simulink model "Pacemaker_Assignment2_group33_Final"  (R2020a)
settings: Solver=FixedStepAuto  StartTime=0.0  StopTime=10.0  FixedStep=1e-3  RelTol=1e-3  EnableMultiTasking=on
undefined symbols (not defined in the file): A0, A1, D0, D1, D10, D11, D12, D13, D2, D3, D4, D5, D6, D7, D8, D9, magnitude, PTA0, PTA1, PTA2, PTB2, PTB23, PTB3, PTB9, PTC16, PTC17, PTC2, PTC3, PTC4, PTD0, PTD1, PTD2, PTD3
libraries: frdmk64flib x22, etargetslib x16, dspstat3 x1
settings Model: ExtModeTrigDuration=5  Creator=sxj  LastModifiedBy=sxj
settings OptimizationCC: EnhancedBackFolding=on  PassReuseOutputArgsAs=Individual arguments  ZeroExternalMemoryAtStartup=off  ZeroInternalMemoryAtStartup=off  MaxStackSize=64  OptimizeBlockOrder=speed  DifferentSizesBufferReuse=on  OptimizationCustomize=off  EfficientTunableParamExpr=on
settings DebuggingCC: ParameterTunabilityLossMsg=error
settings HardwareCC: ProdBitPerPointer=32  ProdBitPerSizeT=32  ProdBitPerPtrDiffT=32  ProdLargestAtomicInteger=Long  ProdLargestAtomicFloat=Double  ProdWordSize=32  ProdHWDeviceType=ARM Compatible->ARM Cortex
settings SFSimCC: MATLABDynamicMemAlloc=off
settings RTWCC: SystemTargetFile=ert.tlc  HardwareBoard=NXP FRDM-K64F  TemplateMakefile=ert_default_tmf  Toolchain=GNU Tools for ARM Embedded Processors
settings CodeAppCC: ForceParamTrailComments=on  IgnoreCustomStorageClasses=off  OperatorAnnotations=on  SimulinkDataObjDesc=on  SFDataObjDesc=on  InsertBlockDesc=on

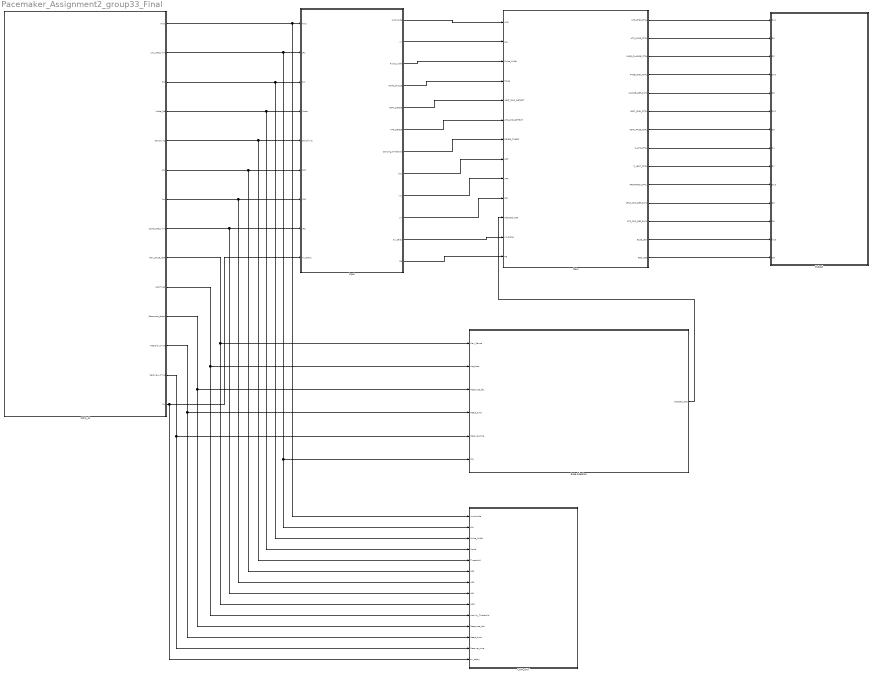
== system Pacemaker_Assignment2_group33_Final ==
  COM_IN : Subsystem
  COM_OUT : Subsystem
  Input : Subsystem
  Main : Stateflow chart  TreatAsAtomicUnit=on
  Output : Subsystem
  Rate Adaption : Subsystem
  wires:
  Input/1(Amplitude) -> Main/1(AMP)
  Input/2(lrl) -> Main/2(LRL)
  Input/3(Pulse_width) -> Main/3(Pulse_Width)
  Input/4(Mode_choose) -> Main/4(Mode)
  Input/5(VENT_SENSE) -> Main/5(VENT_CMP_DETECT)
  Input/6(ATR_SENSE) -> Main/6(ATR_CMP_DETECT)
  Input/7(Sensing_Threshold) -> Main/7(SENSE_THRES)
  Main/1(ATR_GND_CTRL) -> Output/1(D11)
  Main/2(ATR_PACE_CTRL) -> Output/2(D8)
  Main/3(PACE_CHARGE_CTRL) -> Output/3(D2)
  Main/4(PACE_GND_CTRL) -> Output/4(D10)
  Main/5(PACING_REF_PWM) -> Output/5(D5)
  Main/6(VENT_GND_CTRL) -> Output/6(D12)
  Main/7(VENT_PACE_CTRL) -> Output/7(D9)
  Main/8(Z_ATR_CTRL) -> Output/8(D4)
  Main/9(Z_VENT_CTRL) -> Output/9(D7)
  Main/10(FRONTEND_CTRL) -> Output/10(D13)
  Main/11(VENT_CMP_REF_PWM) -> Output/11(D3)
  Main/12(ATR_CMP_REF_PWM) -> Output/12(D6)
  Main/13(BLUE_LED) -> Output/13(blue)
  Main/14(RED_LED) -> Output/14(red)
  Input/8(arp) -> Main/8(ARP)
  Input/9(vrp) -> Main/9(VRP)
  Input/10(url) -> Main/10(URL)
  Rate Adaption/1(Adapted_rate) -> Main/11(Adapted_rate)
  COM_IN/1(Amp) -> COM_OUT/1(Amplitude), Input/1(Amp)
  COM_IN/2(Low_rate_limit) -> COM_OUT/2(LRL), Rate Adaption/6(LRL), Input/2(LRL)
  COM_IN/3(PW) -> COM_OUT/3(Pulse_Width), Input/3(PW)
  COM_IN/4(Mode_Sel) -> COM_OUT/4(Mode), Input/4(Mode)
  COM_IN/5(Sensitivity) -> COM_OUT/5(Threshold), Input/5(Sensitivity)
  COM_IN/6(Arp) -> COM_OUT/6(ARP), Input/6(ARP)
  COM_IN/7(Vrp) -> COM_OUT/7(VRP), Input/7(VRP)
  COM_IN/8(Upper_rate_limit) -> COM_OUT/8(URL), Input/8(URL)
  COM_IN/9(Max_sense_rate) -> COM_OUT/9(MSR), Rate Adaption/1(Max_Sense)
  COM_IN/10(Act_Thres) -> COM_OUT/10(Activity_Threshold), Rate Adaption/2(Act_thres)
  COM_IN/11(Response_factor) -> COM_OUT/11(Response_Fac), Rate Adaption/3(Response_fac)
  COM_IN/12(Reaction_Time) -> COM_OUT/12(React_time), Rate Adaption/4(React_time)
  COM_IN/13(Recovery_Time) -> COM_OUT/13(Recover_time), Rate Adaption/5(Recover_time)
  COM_IN/14(AV) -> COM_OUT/14(av_delay), Input/9(AV_Delay)
  Input/11(av_delay) -> Main/12(AV_Delay)
  Input/12(PB) -> Main/13(PB)

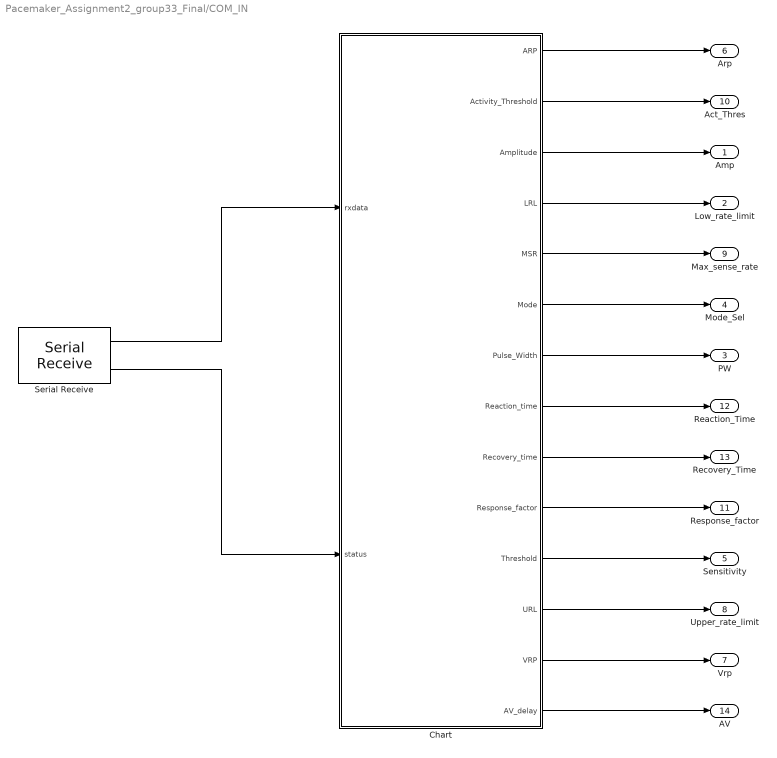
== system Pacemaker_Assignment2_group33_Final/COM_IN ==
  Chart : Stateflow chart  TreatAsAtomicUnit=on
  Serial Receive : frdmk64flib/Serial Receive  SCIModule=0  Baudrate=uint32(9600)  Parity=None  StopBits=1  HardwareFlowControl=None  ByteOrder=LittleEndian  DataType=uint8  DataLength=36  BlockingMode=off  OutputStatus=on  SampleTime=-1
  Amp : Outport
  Low_rate_limit : Outport  Port=2  OutDataTypeStr=uint16
  PW : Outport  Port=3
  Mode_Sel : Outport  Port=4
  Sensitivity : Outport  Port=5
  Arp : Outport  Port=6
  Vrp : Outport  Port=7
  Upper_rate_limit : Outport  Port=8
  Max_sense_rate : Outport  Port=9
  Act_Thres : Outport  Port=10
  Response_factor : Outport  Port=11
  Reaction_Time : Outport  Port=12
  Recovery_Time : Outport  Port=13
  AV : Outport  Port=14
  wires:
  Serial Receive/1 -> Chart/1(rxdata)
  Chart/1(ARP) -> Arp/1
  Chart/2(Activity_Threshold) -> Act_Thres/1
  Chart/3(Amplitude) -> Amp/1
  Chart/4(LRL) -> Low_rate_limit/1
  Chart/5(MSR) -> Max_sense_rate/1
  Chart/6(Mode) -> Mode_Sel/1
  Chart/7(Pulse_Width) -> PW/1
  Chart/8(Reaction_time) -> Reaction_Time/1
  Chart/9(Recovery_time) -> Recovery_Time/1
  Chart/10(Response_factor) -> Response_factor/1
  Chart/11(Threshold) -> Sensitivity/1
  Chart/12(URL) -> Upper_rate_limit/1
  Chart/13(VRP) -> Vrp/1
  Serial Receive/2 -> Chart/2(status)
  Chart/14(AV_delay) -> AV/1

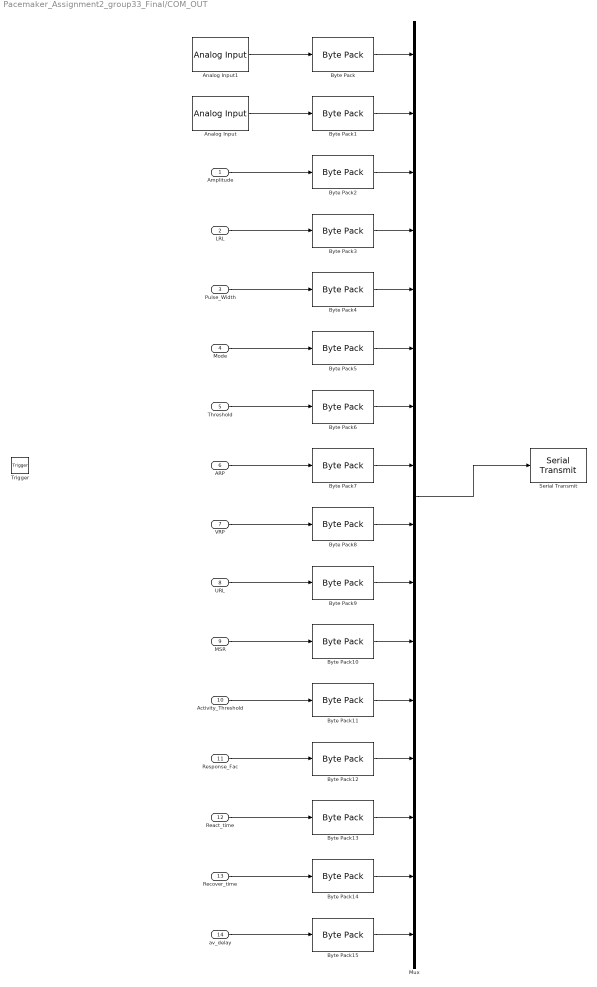
== system Pacemaker_Assignment2_group33_Final/COM_OUT ==
  Amplitude : Inport
  LRL : Inport  Port=2
  Pulse_Width : Inport  Port=3
  Mode : Inport  Port=4
  Threshold : Inport  Port=5
  ARP : Inport  Port=6
  VRP : Inport  Port=7
  URL : Inport  Port=8
  MSR : Inport  Port=9
  Activity_Threshold : Inport  Port=10
  Response_Fac : Inport  Port=11
  React_time : Inport  Port=12
  Recover_time : Inport  Port=13
  av_delay : Inport  Port=14
  Trigger : TriggerPort  TriggerType=function-call  IsSimulinkFunction=on  FunctionName=send_params  VariantControl=Variant  PortDimensions=1
  Analog Input : frdmk64flib/Analog Input  Whichpin=PTB3 (A1)  SampleTime=-1
  Analog Input1 : frdmk64flib/Analog Input  Whichpin=PTB2 (A0)  SampleTime=-1
  Byte Pack : etargetslib/Byte Pack  datatypes={'double'}  byteAlign=1
  Byte Pack1 : etargetslib/Byte Pack  datatypes={'double'}  byteAlign=1
  Byte Pack{2..3,5..6,9..10,12..14} (9 alike) : etargetslib/Byte Pack  datatypes={'uint16'}  byteAlign=1
  Byte Pack{4,7..8,11,15} (5 alike) : etargetslib/Byte Pack  datatypes={'single'}  byteAlign=1
  Mux : Mux  Inputs=16
  Serial Transmit : frdmk64flib/Serial Transmit  SCIModule=0  Baudrate=uint32(9600)  Parity=None  StopBits=1  HardwareFlowControl=None  ByteOrder=LittleEndian  BlockingMode=on  OutputStatus=off
  wires:
  Analog Input/1 -> Byte Pack1/1
  Byte Pack/1 -> Mux/1
  Mux/1 -> Serial Transmit/1
  Analog Input1/1 -> Byte Pack/1
  Byte Pack1/1 -> Mux/2
  LRL/1 -> Byte Pack3/1
  Amplitude/1 -> Byte Pack2/1
  Pulse_Width/1 -> Byte Pack4/1
  Mode/1 -> Byte Pack5/1
  Threshold/1 -> Byte Pack6/1
  ARP/1 -> Byte Pack7/1
  VRP/1 -> Byte Pack8/1
  URL/1 -> Byte Pack9/1
  MSR/1 -> Byte Pack10/1
  Activity_Threshold/1 -> Byte Pack11/1
  Response_Fac/1 -> Byte Pack12/1
  React_time/1 -> Byte Pack13/1
  Recover_time/1 -> Byte Pack14/1
  Byte Pack2/1 -> Mux/3
  Byte Pack3/1 -> Mux/4
  Byte Pack4/1 -> Mux/5
  Byte Pack5/1 -> Mux/6
  Byte Pack6/1 -> Mux/7
  Byte Pack7/1 -> Mux/8
  Byte Pack8/1 -> Mux/9
  Byte Pack9/1 -> Mux/10
  Byte Pack10/1 -> Mux/11
  Byte Pack11/1 -> Mux/12
  Byte Pack12/1 -> Mux/13
  Byte Pack13/1 -> Mux/14
  Byte Pack14/1 -> Mux/15
  av_delay/1 -> Byte Pack15/1
  Byte Pack15/1 -> Mux/16

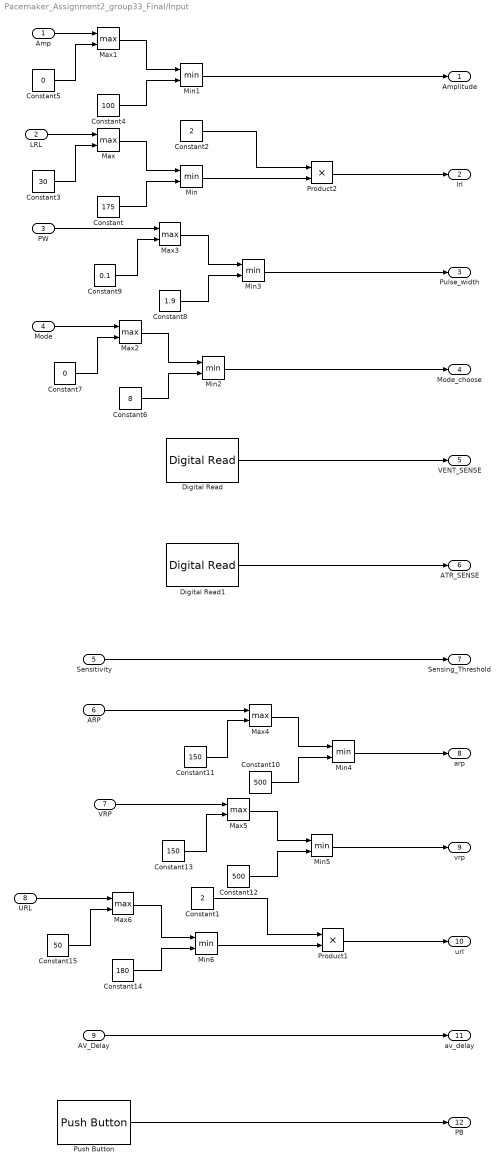
== system Pacemaker_Assignment2_group33_Final/Input ==
  Amp : Inport
  LRL : Inport  Port=2
  PW : Inport  Port=3
  Mode : Inport  Port=4
  Sensitivity : Inport  Port=5
  ARP : Inport  Port=6
  VRP : Inport  Port=7
  URL : Inport  Port=8
  AV_Delay : Inport  Port=9
  Constant : Constant  Value=175
  Constant1 : Constant  Value=2
  Constant10 : Constant  Value=500
  Constant11 : Constant  Value=150
  Constant12 : Constant  Value=500
  Constant13 : Constant  Value=150
  Constant14 : Constant  Value=180
  Constant15 : Constant  Value=50
  Constant2 : Constant  Value=2
  Constant3 : Constant  Value=30
  Constant4 : Constant  Value=100
  Constant5 : Constant  Value=0
  Constant6 : Constant  Value=8
  Constant7 : Constant  Value=0
  Constant8 : Constant  Value=1.9
  Constant9 : Constant  Value=0.1
  Digital Read : frdmk64flib/Digital Read  Whichpin=PTC17 (D1)  SampleTime=-1
  Digital Read1 : frdmk64flib/Digital Read  Whichpin=PTC16 (D0)  SampleTime=-1
  Max{,3..5} (4 alike) : MinMax  Function=max  Inputs=2  OutDataTypeStr=single
  Max1 : MinMax  Function=max  Inputs=2  OutDataTypeStr=uint16
  Max2 : MinMax  Function=max  Inputs=2  OutDataTypeStr=uint16
  Max6 : MinMax  Function=max  Inputs=2
  Min{,3..5} (4 alike) : MinMax  Inputs=2  OutDataTypeStr=single
  Min1 : MinMax  Inputs=2  OutDataTypeStr=uint16
  Min2 : MinMax  Inputs=2  OutDataTypeStr=uint16
  Min6 : MinMax  Inputs=2
  Product1 : Product  OutDataTypeStr=uint16
  Product2 : Product  OutDataTypeStr=single
  Push Button : frdmk64flib/Push Button  Whichswitch=SW2  SampleTime1=-1
  Amplitude : Outport
  lrl : Outport  Port=2
  Pulse_width : Outport  Port=3
  Mode_choose : Outport  Port=4
  VENT_SENSE : Outport  Port=5
  ATR_SENSE : Outport  Port=6
  Sensing_Threshold : Outport  Port=7
  arp : Outport  Port=8
  vrp : Outport  Port=9
  url : Outport  Port=10
  av_delay : Outport  Port=11
  PB : Outport  Port=12
  wires:
  Digital Read/1 -> VENT_SENSE/1
  Digital Read1/1 -> ATR_SENSE/1
  Sensitivity/1 -> Sensing_Threshold/1
  Product1/1 -> url/1
  Constant1/1 -> Product1/1
  Constant2/1 -> Product2/1
  Product2/1 -> lrl/1
  AV_Delay/1 -> av_delay/1
  Push Button/1 -> PB/1
  Constant/1 -> Min/2
  Max/1 -> Min/1
  Constant3/1 -> Max/2
  Min/1 -> Product2/2
  Constant4/1 -> Min1/2
  Constant5/1 -> Max1/2
  Max1/1 -> Min1/1
  Amp/1 -> Max1/1
  LRL/1 -> Max/1
  Min1/1 -> Amplitude/1
  Constant6/1 -> Min2/2
  Constant7/1 -> Max2/2
  Max2/1 -> Min2/1
  Min2/1 -> Mode_choose/1
  Mode/1 -> Max2/1
  Constant8/1 -> Min3/2
  Constant9/1 -> Max3/2
  Max3/1 -> Min3/1
  PW/1 -> Max3/1
  Min3/1 -> Pulse_width/1
  Constant10/1 -> Min4/2
  Constant11/1 -> Max4/2
  Max4/1 -> Min4/1
  Min4/1 -> arp/1
  ARP/1 -> Max4/1
  Constant12/1 -> Min5/2
  Constant13/1 -> Max5/2
  Max5/1 -> Min5/1
  Min5/1 -> vrp/1
  VRP/1 -> Max5/1
  Constant14/1 -> Min6/2
  Constant15/1 -> Max6/2
  Max6/1 -> Min6/1
  Min6/1 -> Product1/2
  URL/1 -> Max6/1

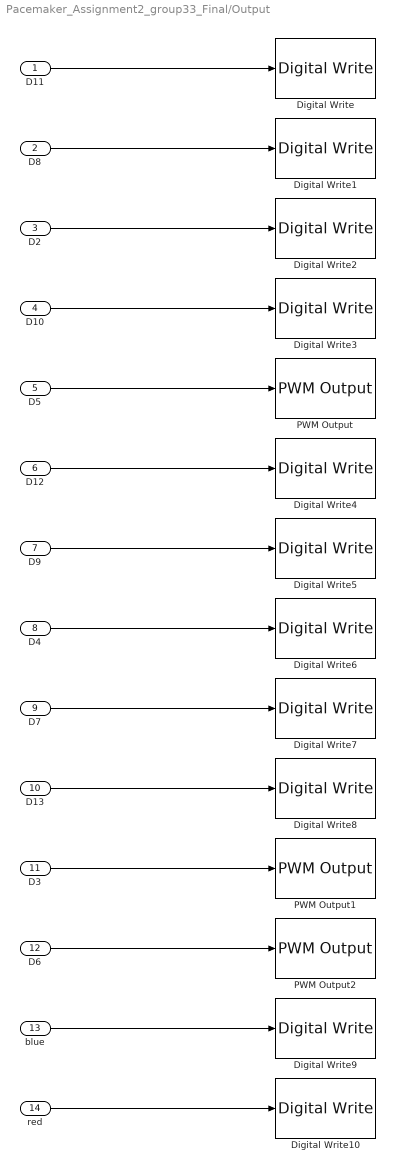
== system Pacemaker_Assignment2_group33_Final/Output ==
  D11 : Inport
  D8 : Inport  Port=2
  D2 : Inport  Port=3
  D10 : Inport  Port=4
  D5 : Inport  Port=5
  D12 : Inport  Port=6
  D9 : Inport  Port=7
  D4 : Inport  Port=8
  D7 : Inport  Port=9
  D13 : Inport  Port=10
  D3 : Inport  Port=11
  D6 : Inport  Port=12
  blue : Inport  Port=13
  red : Inport  Port=14
  Digital Write : frdmk64flib/Digital Write  Whichpin=PTD2 (D11)
  Digital Write1 : frdmk64flib/Digital Write  Whichpin=PTA0 (D8)
  Digital Write10 : frdmk64flib/Digital Write  Whichpin=RED_LED
  Digital Write2 : frdmk64flib/Digital Write  Whichpin=PTB9 (D2)
  Digital Write3 : frdmk64flib/Digital Write  Whichpin=PTD0 (D10)
  Digital Write4 : frdmk64flib/Digital Write  Whichpin=PTD3 (D12)
  Digital Write5 : frdmk64flib/Digital Write  Whichpin=PTC4 (D9)
  Digital Write6 : frdmk64flib/Digital Write  Whichpin=PTB23 (D4)
  Digital Write7 : frdmk64flib/Digital Write  Whichpin=PTC3 (D7)
  Digital Write8 : frdmk64flib/Digital Write  Whichpin=PTD1 (D13)
  Digital Write9 : frdmk64flib/Digital Write  Whichpin=BLUE_LED
  PWM Output : frdmk64flib/PWM Output  Whichpin=PTA2 (D5)  InitialFrequency=2000  InitialDutyCycle=0
  PWM Output1 : frdmk64flib/PWM Output  Whichpin=PTA1 (D3)  InitialFrequency=2000  InitialDutyCycle=0
  PWM Output2 : frdmk64flib/PWM Output  Whichpin=PTC2 (D6)  InitialFrequency=2000  InitialDutyCycle=0
  wires:
  D11/1 -> Digital Write/1
  D8/1 -> Digital Write1/1
  D2/1 -> Digital Write2/1
  D10/1 -> Digital Write3/1
  D5/1 -> PWM Output/1
  D12/1 -> Digital Write4/1
  D9/1 -> Digital Write5/1
  D4/1 -> Digital Write6/1
  D7/1 -> Digital Write7/1
  D13/1 -> Digital Write8/1
  D3/1 -> PWM Output1/1
  D6/1 -> PWM Output2/1
  blue/1 -> Digital Write9/1
  red/1 -> Digital Write10/1

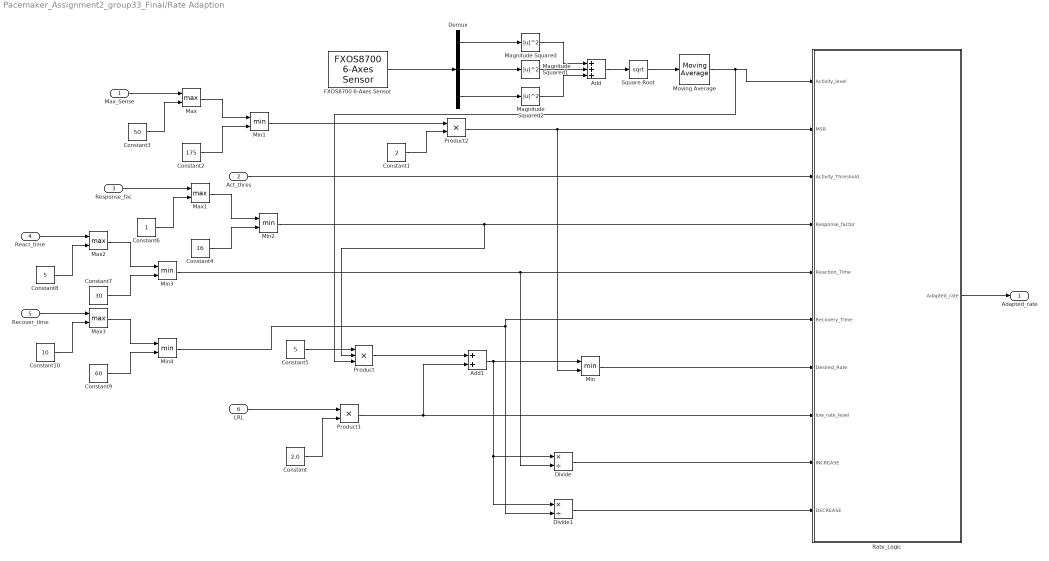
== system Pacemaker_Assignment2_group33_Final/Rate Adaption ==
  Max_Sense : Inport
  Act_thres : Inport  Port=2
  Response_fac : Inport  Port=3
  React_time : Inport  Port=4
  Recover_time : Inport  Port=5
  LRL : Inport  Port=6  OutDataTypeStr=uint16
  Add : Sum  Inputs=+++
  Add1 : Sum
  Constant : Constant  Value=2.0
  Constant1 : Constant  Value=2
  Constant10 : Constant  Value=10
  Constant2 : Constant  Value=175
  Constant3 : Constant  Value=50
  Constant4 : Constant  Value=16
  Constant5 : Constant  Value=5
  Constant6 : Constant
  Constant7 : Constant  Value=30
  Constant8 : Constant  Value=5
  Constant9 : Constant  Value=60
  Demux : Demux  Outputs=3
  Divide : Product  Inputs=*/
  Divide1 : Product  Inputs=*/
  FXOS8700 6-Axes Sensor : frdmk64flib/FXOS8700 6-Axes Sensor  Activesensor=Accelerometer only  ODR=800Hz  HybridODR=400Hz  Accelfullrange=-4g to +4g  SampleTime=-1
  Magnitude Squared : Math  Operator=magnitude^2  SaturateOnIntegerOverflow=on
  Magnitude Squared1 : Math  Operator=magnitude^2  SaturateOnIntegerOverflow=on
  Magnitude Squared2 : Math  Operator=magnitude^2  SaturateOnIntegerOverflow=on
  Max{,1..3} (4 alike) : MinMax  Function=max  Inputs=2  OutDataTypeStr=uint16
  Min : MinMax  Inputs=2
  Min{1..4} (4 alike) : MinMax  Inputs=2  OutDataTypeStr=uint16
  Moving Average : dspstat3/Moving Average  Method=Sliding window  ForgettingFactorPort=off  SpecifyWindowLength=on  WindowLength=100  ForgettingFactor=0.9  SimulateUsing=Code generation
  Product : Product  Inputs=3
  Product1 : Product  OutDataTypeStr=double
  Product2 : Product  OutDataTypeStr=uint8
  Rate_Logic : Stateflow chart  TreatAsAtomicUnit=on
  Square Root : Sqrt  SaturateOnIntegerOverflow=on
  Adapted_rate : Outport
  wires:
  Demux/1 -> Magnitude Squared/1
  Magnitude Squared1/1 -> Add/2
  Add/1 -> Square Root/1
  FXOS8700 6-Axes Sensor/1 -> Demux/1
  Demux/2 -> Magnitude Squared1/1
  Demux/3 -> Magnitude Squared2/1
  Magnitude Squared/1 -> Add/1
  Magnitude Squared2/1 -> Add/3
  Square Root/1 -> Moving Average/1
  Min2/1 -> Product/2, Rate_Logic/4(Response_factor)
  Min3/1 -> Rate_Logic/5(Reaction_Time), Divide/2
  Min4/1 -> Rate_Logic/6(Recovery_Time), Divide1/2
  Moving Average/1 -> Product/3, Rate_Logic/1(Activity_level)
  Product/1 -> Add1/1
  Product1/1 -> Add1/2, Rate_Logic/8(low_rate_level)
  Add1/1 -> Divide1/1, Divide/1, Min/1
  Min/1 -> Rate_Logic/7(Desired_Rate)
  Divide/1 -> Rate_Logic/9(INCREASE)
  Rate_Logic/1(Adapted_rate) -> Adapted_rate/1
  Constant5/1 -> Product/1
  Divide1/1 -> Rate_Logic/10(DECREASE)
  LRL/1 -> Product1/1
  Product2/1 -> Min/2, Rate_Logic/2(MSR)
  Act_thres/1 -> Rate_Logic/3(Activity_Threshold)
  Constant/1 -> Product1/2
  Constant1/1 -> Product2/2
  Constant2/1 -> Min1/2
  Constant3/1 -> Max/2
  Max/1 -> Min1/1
  Min1/1 -> Product2/1
  Max_Sense/1 -> Max/1
  Constant4/1 -> Min2/2
  Constant6/1 -> Max1/2
  Max1/1 -> Min2/1
  Response_fac/1 -> Max1/1
  Constant7/1 -> Min3/2
  Constant8/1 -> Max2/2
  Max2/1 -> Min3/1
  React_time/1 -> Max2/1
  Constant9/1 -> Min4/2
  Constant10/1 -> Max3/2
  Max3/1 -> Min4/1
  Recover_time/1 -> Max3/1

== stateflow chart Pacemaker_Assignment2_group33_Final/Rate Adaption/Rate_Logic ==
  state Increase_pend
  state Initialize
    entry:
    Adapted_rate = low_rate_level;
  state Increase_
    entry:
    Adapted_rate = Adapted_rate + INCREASE;
  state Reached_desire
    entry:
    Adapted_rate = Desired_Rate;
  state Inc_Dec
  state Dec_Inc
  state Decrease_
    entry:
    Adapted_rate = Adapted_rate - DECREASE;
  state Decrease_pend
  Increase_pend -> Increase_ : after(Reaction_Time,msec)
  Increase_ -> Increase_pend [order 1] : [Adapted_rate < Desired_Rate]
  (default) -> Initialize
  Initialize -> Initialize [order 2] : [Activity_level <= Activity_Threshold]
  Reached_desire -> Reached_desire [order 2] : [Activity_level > Activity_Threshold]
  Initialize -> Increase_ [order 1] : [Activity_level > Activity_Threshold]
  Increase_ -> Reached_desire [order 2] : [Adapted_rate >= Desired_Rate]
  Increase_ -> Inc_Dec [order 3] : [Activity_level <= Activity_Threshold]
  Dec_Inc -> Increase_ : after(Reaction_Time,msec)
  Decrease_ -> Initialize [order 2] : [Adapted_rate <= low_rate_level]
  Reached_desire -> Decrease_ [order 1] : [Activity_level <= Activity_Threshold]
  Inc_Dec -> Decrease_ : after(Recovery_Time,msec)
  Decrease_ -> Dec_Inc [order 1] : [Activity_level > Activity_Threshold]
  Decrease_ -> Decrease_pend [order 3] : [Adapted_rate > low_rate_level]
  Decrease_pend -> Decrease_ : after(Recovery_Time,msec)
  data: Activity_level input; MSR input uint8; Activity_Threshold input single; Response_factor input uint16; Reaction_Time input uint16; Recovery_Time input uint16; Desired_Rate input; low_rate_level input double; INCREASE input; DECREASE input; Adapted_rate output double

== stateflow chart Pacemaker_Assignment2_group33_Final/COM_IN/Chart ==
  state SEND_PARAM
    entry:
    Mode =typecast(rxdata(3:4),'uint16');
    Amplitude = typecast(rxdata(5:6),'uint16');
    LRL = typecast(rxdata(7:8),'uint16');
    Pulse_Width = typecast(rxdata(9:12),'single');
    Threshold = typecast(rxdata(13:14),'uint16');
    ARP = typecast(rxdata(15:18),'single');
    VRP = typecast(rxdata(19:22),'single');
    URL = typecast(rxdata(23:24),'uint16');
    MSR = typecast(rxdata(25:26),'uint16');
    Activity_Threshold = typecast(rxdata(27:30),'single');
    Response_factor = typecast(rxdata(31:32),'uint16');
    Reaction_time = typecast(rxdata(33:34),'uint16');
    Recovery_time = typecast(rxdata(35:36),'uint16');
    AV_delay = typecast(rxdata(37:40),'single');
  state Initial_State
    entry:
    Mode = 4;
    Amplitude = 100;
    LRL = 60;
    Pulse_Width = 0.4; %4/10 = 0.4
    Threshold = 66;
    ARP = 320; %2 byte
    VRP = 320; %2 byte
    URL = 120; %2 byte
    MSR = 120; %2 byte
    Activity_Threshold = 1.1; %11/10 = 1.1
    Response_factor = 8;
    Reaction_time = 10;
    Recovery_time = 30;
    AV_delay = 150;
  state STANDBY
  state SEND_BACK
    entry:
    send_params();
  SEND_PARAM -> STANDBY
  (junction 10) -> SEND_PARAM [order 1] : [rxdata(2) == hex2dec('55')]
  (default) -> Initial_State
  (junction 7) -> STANDBY [order 2]
  Initial_State -> STANDBY
  STANDBY -> (junction 7) : [status == 0]
  (junction 7) -> (junction 10) [order 1] : [rxdata(1) == hex2dec('16')]
  (junction 10) -> SEND_BACK [order 2] : [rxdata(2) == hex2dec('22')]
  SEND_BACK -> STANDBY
  data: rxdata input uint8; status input uint8; ARP output single; Activity_Threshold output single; Amplitude output uint16; LRL output uint16; MSR output uint16; Mode output uint16; Pulse_Width output single; Reaction_time output uint16; Recovery_time output uint16; Response_factor output uint16; Threshold output uint16; URL output uint16; VRP output single; AV_delay output single

== stateflow chart Pacemaker_Assignment2_group33_Final/Main ==
  state AOO
    state AOO_CHARGE
      %State for charging C22 and Discharging C21
      entry:
      PACING_REF_PWM = AMP;
      PACE_CHARGE_CTRL = 1;
      ATR_PACE_CTRL = 0;
      ATR_GND_CTRL = 1;
      PACE_GND_CTRL = 1;
      Z_ATR_CTRL = 0;
      VENT_PACE_CTRL = 0;
      VENT_GND_CTRL = 0;
      Z_VENT_CTRL = 0;
      BLUE_LED = 1;
      RED_LED = 0;
    state AOO_PACE
      %State for pacemaker actual pacing
      entry:
      PACING_REF_PWM = AMP;
      PACE_CHARGE_CTRL = 0;
      ATR_PACE_CTRL = 1;
      ATR_GND_CTRL = 0;
      PACE_GND_CTRL = 1;
      Z_ATR_CTRL = 0;
      VENT_PACE_CTRL = 0;
      VENT_GND_CTRL = 0;
      Z_VENT_CTRL = 0;
      BLUE_LED = 1;
      RED_LED = 0;
    (default) -> AOO_CHARGE
    AOO_CHARGE -> AOO_PACE : [after(60000/LRL-Pulse_Width,msec)]
    AOO_PACE -> AOO_CHARGE : [after(Pulse_Width,msec)]
  state AOOR
    state AOOR_PACE
      %State for pacemaker actual pacing
      entry:
      PACING_REF_PWM = AMP;
      PACE_CHARGE_CTRL = 0;
      ATR_PACE_CTRL = 1;
      ATR_GND_CTRL = 0;
      PACE_GND_CTRL = 1;
      Z_ATR_CTRL = 0;
      VENT_PACE_CTRL = 0;
      VENT_GND_CTRL = 0;
      Z_VENT_CTRL = 0;
      BLUE_LED = 1;
      RED_LED = 0;
    state AOOR_CHARGE
      %State for charging C22 and Discharging C21
      entry:
      PACING_REF_PWM = AMP;
      PACE_CHARGE_CTRL = 1;
      ATR_PACE_CTRL = 0;
      ATR_GND_CTRL = 1;
      PACE_GND_CTRL = 1;
      Z_ATR_CTRL = 0;
      VENT_PACE_CTRL = 0;
      VENT_GND_CTRL = 0;
      Z_VENT_CTRL = 0;
      BLUE_LED = 0;
      RED_LED = 1;
    (default) -> AOOR_CHARGE
    AOOR_CHARGE -> AOOR_PACE : after(60000/Adapted_rate-Pulse_Width,msec)
    AOOR_PACE -> AOOR_CHARGE : after(Pulse_Width,msec)
  state VVIR
    state VVI_entry
      %Entry State setting variables
      % identical to Charging State
      entry:
      PACING_REF_PWM = AMP;
      PACE_CHARGE_CTRL = 1;
      VENT_PACE_CTRL = 0;
      VENT_GND_CTRL = 1;
      PACE_GND_CTRL = 1;
      Z_VENT_CTRL = 0;
      FRONTEND_CTRL = 1;
      VENT_CMP_REF_PWM = SENSE_THRES;
      ATR_PACE_CTRL = 0;
      ATR_GND_CTRL = 0;
      Z_ATR_CTRL = 0;
    state Sensed
      %Natural activities detected
    state VVI_CHARGE
      %State for charging C22 and Discharging C21
      entry:
      PACING_REF_PWM = AMP;
      PACE_CHARGE_CTRL = 1;
      VENT_PACE_CTRL = 0;
      VENT_GND_CTRL = 1;
      PACE_GND_CTRL = 1;
      Z_VENT_CTRL = 0;
      FRONTEND_CTRL = 1;
      VENT_CMP_REF_PWM = SENSE_THRES;
      ATR_PACE_CTRL = 0;
      ATR_GND_CTRL = 0;
      Z_ATR_CTRL = 0;
    state VVI_Sense
      %Detect Natural activities
    state VVI_PACE
      %State for pacamekr actual pacing
      entry:
      PACING_REF_PWM = AMP;
      PACE_CHARGE_CTRL = 0;
      VENT_PACE_CTRL = 1;
      VENT_GND_CTRL = 0;
      PACE_GND_CTRL = 1;
      Z_VENT_CTRL = 0;
      FRONTEND_CTRL = 1;
      VENT_CMP_REF_PWM = SENSE_THRES;
      ATR_PACE_CTRL = 0;
      ATR_GND_CTRL = 0;
      Z_ATR_CTRL = 0;
    (default) -> VVIR.VVI_entry
    VVIR.Sensed -> VVIR.VVI_Sense : after(VRP,msec)
    VVIR.VVI_entry -> VVIR.VVI_Sense
    VVIR.VVI_Sense -> VVIR.Sensed [order 1] : [VENT_CMP_DETECT == 1]
    VVIR.VVI_Sense -> VVIR.VVI_PACE [order 2] : after((60000/Adapted_rate)-VRP,msec)
    VVIR.VVI_CHARGE -> VVIR.VVI_Sense : after(VRP-Pulse_Width,msec)
    VVIR.VVI_PACE -> VVIR.VVI_CHARGE : after(Pulse_Width,msec)
  state IDLE_STATE
  state VVI
    state VVI_entry
      %Entry State setting variables
      % identical to Charging State
      entry:
      PACING_REF_PWM = AMP;
      PACE_CHARGE_CTRL = 1;
      VENT_PACE_CTRL = 0;
      VENT_GND_CTRL = 1;
      PACE_GND_CTRL = 1;
      Z_VENT_CTRL = 0;
      FRONTEND_CTRL = 1;
      VENT_CMP_REF_PWM = SENSE_THRES;
      ATR_PACE_CTRL = 0;
      ATR_GND_CTRL = 0;
      Z_ATR_CTRL = 0;
    state Sensed
      %Natural activities detected
    state VVI_CHARGE
      %State for charging C22 and Discharging C21
      entry:
      PACING_REF_PWM = AMP;
      PACE_CHARGE_CTRL = 1;
      VENT_PACE_CTRL = 0;
      VENT_GND_CTRL = 1;
      PACE_GND_CTRL = 1;
      Z_VENT_CTRL = 0;
      FRONTEND_CTRL = 1;
      VENT_CMP_REF_PWM = SENSE_THRES;
      ATR_PACE_CTRL = 0;
      ATR_GND_CTRL = 0;
      Z_ATR_CTRL = 0;
    state VVI_Sense
      %Detect Natural activities
    state VVI_PACE
      %State for pacamekr actual pacing
      entry:
      PACING_REF_PWM = AMP;
      PACE_CHARGE_CTRL = 0;
      VENT_PACE_CTRL = 1;
      VENT_GND_CTRL = 0;
      PACE_GND_CTRL = 1;
      Z_VENT_CTRL = 0;
      FRONTEND_CTRL = 1;
      VENT_CMP_REF_PWM = SENSE_THRES;
      ATR_PACE_CTRL = 0;
      ATR_GND_CTRL = 0;
      Z_ATR_CTRL = 0;
    (default) -> VVI.VVI_entry
    VVI.Sensed -> VVI.VVI_Sense : after(VRP,msec)
    VVI.VVI_entry -> VVI.VVI_Sense
    VVI.VVI_Sense -> VVI.Sensed [order 1] : [VENT_CMP_DETECT == 1]
    VVI.VVI_Sense -> VVI.VVI_PACE [order 2] : after((60000/LRL)-VRP,msec)
    VVI.VVI_CHARGE -> VVI.VVI_Sense : after(VRP-Pulse_Width,msec)
    VVI.VVI_PACE -> VVI.VVI_CHARGE : after(Pulse_Width,msec)
  state AAI
    state AAI_entry
      %Entry State setting variables
      % identical to Charging State
      entry:
      PACING_REF_PWM = AMP;
      PACE_CHARGE_CTRL = 1;
      ATR_PACE_CTRL = 0;
      ATR_GND_CTRL = 1;
      PACE_GND_CTRL = 1;
      Z_ATR_CTRL = 0;
      FRONTEND_CTRL = 1;
      ATR_CMP_REF_PWM = SENSE_THRES;
      VENT_PACE_CTRL = 0;
      VENT_GND_CTRL = 0;
      Z_VENT_CTRL = 0;
    state AAI_Sensed
      %Nastural actvites Detected
    state AAI_PACE
      %State for pacamekr actual pacing
      entry:
      PACING_REF_PWM = AMP;
      PACE_CHARGE_CTRL = 0;
      ATR_PACE_CTRL = 1;
      ATR_GND_CTRL = 0;
      PACE_GND_CTRL = 1;
      Z_ATR_CTRL = 0;
      FRONTEND_CTRL = 1;
      ATR_CMP_REF_PWM = SENSE_THRES;
      VENT_PACE_CTRL = 0;
      VENT_GND_CTRL = 0;
      Z_VENT_CTRL = 0;
    state AAI_CHARGE
      %State for charging C22 and Discharging C21
      entry:
      PACING_REF_PWM = AMP;
      PACE_CHARGE_CTRL = 1;
      ATR_PACE_CTRL = 0;
      ATR_GND_CTRL = 1;
      PACE_GND_CTRL = 1;
      Z_ATR_CTRL = 0;
      FRONTEND_CTRL = 1;
      ATR_CMP_REF_PWM = SENSE_THRES;
      VENT_PACE_CTRL = 0;
      VENT_GND_CTRL = 0;
      Z_VENT_CTRL = 0;
    state AAI_Sense
      %Detect Natural activities
    (default) -> AAI.AAI_entry
    AAI.AAI_entry -> AAI.AAI_Sense
    AAI.AAI_Sensed -> AAI.AAI_Sense : after(ARP,msec)
    AAI.AAI_Sense -> AAI.AAI_Sensed [order 1] : [ATR_CMP_DETECT == 1]
    AAI.AAI_CHARGE -> AAI.AAI_Sense : after(ARP-Pulse_Width,msec)
    AAI.AAI_Sense -> AAI.AAI_PACE [order 2] : after((60000/LRL)-ARP,msec)
    AAI.AAI_PACE -> AAI.AAI_CHARGE : after(Pulse_Width,msec)
  state AAIR
    state AAI_entry
      %Entry State setting variables
      % identical to Charging State
      entry:
      PACING_REF_PWM = AMP;
      PACE_CHARGE_CTRL = 1;
      ATR_PACE_CTRL = 0;
      ATR_GND_CTRL = 1;
      PACE_GND_CTRL = 1;
      Z_ATR_CTRL = 0;
      FRONTEND_CTRL = 1;
      ATR_CMP_REF_PWM = SENSE_THRES;
      VENT_PACE_CTRL = 0;
      VENT_GND_CTRL = 0;
      Z_VENT_CTRL = 0;
    state AAI_Sensed
      %Nastural actvites Detected
    state AAI_PACE
      %State for pacamekr actual pacing
      entry:
      PACING_REF_PWM = AMP;
      PACE_CHARGE_CTRL = 0;
      ATR_PACE_CTRL = 1;
      ATR_GND_CTRL = 0;
      PACE_GND_CTRL = 1;
      Z_ATR_CTRL = 0;
      FRONTEND_CTRL = 1;
      ATR_CMP_REF_PWM = SENSE_THRES;
      VENT_PACE_CTRL = 0;
      VENT_GND_CTRL = 0;
      Z_VENT_CTRL = 0;
    state AAI_CHARGE
      %State for charging C22 and Discharging C21
      entry:
      PACING_REF_PWM = AMP;
      PACE_CHARGE_CTRL = 1;
      ATR_PACE_CTRL = 0;
      ATR_GND_CTRL = 1;
      PACE_GND_CTRL = 1;
      Z_ATR_CTRL = 0;
      FRONTEND_CTRL = 1;
      ATR_CMP_REF_PWM = SENSE_THRES;
      VENT_PACE_CTRL = 0;
      VENT_GND_CTRL = 0;
      Z_VENT_CTRL = 0;
    state AAI_Sense
      %Detect Natural activities
    (default) -> AAIR.AAI_entry
    AAIR.AAI_entry -> AAIR.AAI_Sense
    AAIR.AAI_Sensed -> AAIR.AAI_Sense : after(ARP,msec)
    AAIR.AAI_Sense -> AAIR.AAI_Sensed [order 1] : [ATR_CMP_DETECT == 1]
    AAIR.AAI_CHARGE -> AAIR.AAI_Sense : after(ARP-Pulse_Width,msec)
    AAIR.AAI_Sense -> AAIR.AAI_PACE [order 2] : after((60000/Adapted_rate)-ARP,msec)
    AAIR.AAI_PACE -> AAIR.AAI_CHARGE : after(Pulse_Width,msec)
  state VOOR
    state VOO_PACE
      %State for pacemaker actual pacing
      entry:
      PACING_REF_PWM = AMP;
      PACE_CHARGE_CTRL = 0;
      VENT_PACE_CTRL = 1;
      VENT_GND_CTRL = 0;
      PACE_GND_CTRL = 1;
      Z_VENT_CTRL = 0;
      ATR_PACE_CTRL = 0;
      ATR_GND_CTRL = 0;
      Z_ATR_CTRL = 0;
      BLUE_LED = 1;
      RED_LED = 0;
    state VOO_CHARGE
      %State for charging C22 and Discharging C21
      entry:
      PACING_REF_PWM = AMP;
      PACE_CHARGE_CTRL = 1;
      VENT_PACE_CTRL = 0;
      VENT_GND_CTRL = 1;
      PACE_GND_CTRL = 1;
      Z_VENT_CTRL = 0;
      ATR_PACE_CTRL = 0;
      ATR_GND_CTRL = 0;
      Z_ATR_CTRL = 0;
      BLUE_LED = 0;
      RED_LED = 1;
    (default) -> VOOR.VOO_CHARGE
    VOOR.VOO_CHARGE -> VOOR.VOO_PACE : after(60000/Adapted_rate-Pulse_Width,msec)
    VOOR.VOO_PACE -> VOOR.VOO_CHARGE : after(Pulse_Width,msec)
  state VOO
    state VOO_CHARGE
      %State for charging C22 and Discharging C21
      entry:
      PACING_REF_PWM = AMP;
      PACE_CHARGE_CTRL = 1;
      VENT_PACE_CTRL = 0;
      VENT_GND_CTRL = 1;
      PACE_GND_CTRL = 1;
      Z_VENT_CTRL = 0;
      ATR_PACE_CTRL = 0;
      ATR_GND_CTRL = 0;
      Z_ATR_CTRL = 0;
      BLUE_LED = 0;
      RED_LED = 1;
    state VOO_PACE
      %State for pacemaker actual pacing
      entry:
      PACING_REF_PWM = AMP;
      PACE_CHARGE_CTRL = 0;
      VENT_PACE_CTRL = 1;
      VENT_GND_CTRL = 0;
      PACE_GND_CTRL = 1;
      Z_VENT_CTRL = 0;
      ATR_PACE_CTRL = 0;
      ATR_GND_CTRL = 0;
      Z_ATR_CTRL = 0;
      BLUE_LED = 0;
      RED_LED = 1;
    (default) -> VOO.VOO_CHARGE
    VOO.VOO_CHARGE -> VOO.VOO_PACE : after((60000/LRL)-Pulse_Width,msec)
    VOO.VOO_PACE -> VOO.VOO_CHARGE : after(Pulse_Width,msec)
  state DDDR
    state DDDR_entry
      %Entry State setting variables
      entry:
      PACING_REF_PWM = AMP;
      PACE_CHARGE_CTRL = 1;
      ATR_PACE_CTRL = 0;
      ATR_GND_CTRL = 0;
      PACE_GND_CTRL = 1;
      Z_ATR_CTRL = 0;
      FRONTEND_CTRL = 1;
      ATR_CMP_REF_PWM = SENSE_THRES;
      VENT_PACE_CTRL = 0;
      VENT_GND_CTRL = 0;
      Z_VENT_CTRL = 0;
    state Ventricle_Sensing
      %Detect Ventricle activities
    state Atrial_Sensing
      %Detect Atrial activities
    state Atrial_Sensed
      %Detect Atrial activities
    state Ventricle_Sensed1
      %Detected ventricle activities
    state DDDR_charge
      %Entry State setting variables
      entry:
      PACING_REF_PWM = AMP;
      PACE_CHARGE_CTRL = 1;
      ATR_PACE_CTRL = 0;
      ATR_GND_CTRL = 0;
      PACE_GND_CTRL = 1;
      Z_ATR_CTRL = 0;
      FRONTEND_CTRL = 1;
      ATR_CMP_REF_PWM = SENSE_THRES;
      VENT_PACE_CTRL = 0;
      VENT_GND_CTRL = 1;
      Z_VENT_CTRL = 0;
    state DDDR_PaceA
      %Entry State setting variables
      entry:
      PACING_REF_PWM = AMP;
      PACE_CHARGE_CTRL = 0;
      ATR_PACE_CTRL = 1;
      ATR_GND_CTRL = 0;
      PACE_GND_CTRL = 1;
      Z_ATR_CTRL = 0;
      FRONTEND_CTRL = 1;
      ATR_CMP_REF_PWM = SENSE_THRES;
      VENT_PACE_CTRL = 0;
      VENT_GND_CTRL = 0;
      Z_VENT_CTRL = 0;
    state Ventricle_Sensing1
      %Detect Ventricle activities
      entry:
      PACING_REF_PWM = AMP;
      PACE_CHARGE_CTRL = 1;
      ATR_PACE_CTRL = 0;
      ATR_GND_CTRL = 1;
      PACE_GND_CTRL = 1;
      Z_ATR_CTRL = 0;
      FRONTEND_CTRL = 1;
      ATR_CMP_REF_PWM = SENSE_THRES;
      VENT_PACE_CTRL = 0;
      VENT_GND_CTRL = 0;
      Z_VENT_CTRL = 0;
    state Ventricle_Sensed2
      %Detected ventricle activities
    state DDDR_PaceV1
      %Entry State setting variables
      entry:
      PACING_REF_PWM = AMP;
      PACE_CHARGE_CTRL = 0;
      ATR_PACE_CTRL = 0;
      ATR_GND_CTRL = 0;
      PACE_GND_CTRL = 1;
      Z_ATR_CTRL = 0;
      FRONTEND_CTRL = 1;
      ATR_CMP_REF_PWM = SENSE_THRES;
      VENT_PACE_CTRL = 1;
      VENT_GND_CTRL = 0;
      Z_VENT_CTRL = 0;
    state DDDR_PaceV
      %Entry State setting variables
      entry:
      PACING_REF_PWM = AMP;
      PACE_CHARGE_CTRL = 0;
      ATR_PACE_CTRL = 0;
      ATR_GND_CTRL = 0;
      PACE_GND_CTRL = 1;
      Z_ATR_CTRL = 0;
      FRONTEND_CTRL = 1;
      ATR_CMP_REF_PWM = SENSE_THRES;
      VENT_PACE_CTRL = 1;
      VENT_GND_CTRL = 0;
      Z_VENT_CTRL = 0;
    Ventricle_Sensed1 -> DDDR_entry : [after(ARP-AV_Delay,msec)]
    Ventricle_Sensed2 -> DDDR_entry : [after(60000/LRL-AV_Delay,msec)]
    (default) -> DDDR_entry
    Ventricle_Sensing -> Ventricle_Sensed1 [order 2] : [PB == 1]
    Atrial_Sensed -> Ventricle_Sensing : [after(AV_Delay,msec)]
    Atrial_Sensing -> Atrial_Sensed [order 1] : [ATR_CMP_DETECT == 1]
    DDDR_entry -> Atrial_Sensing
    Ventricle_Sensing -> Ventricle_Sensed1 [order 1] : [VENT_CMP_DETECT == 1]
    Ventricle_Sensing -> DDDR_PaceV1 [order 3] : [VENT_CMP_DETECT == 0]
    Atrial_Sensing -> DDDR_PaceA [order 2] : [ATR_CMP_DETECT == 0]
    DDDR_charge -> DDDR_entry : [after(60000/LRL-AV_Delay-Pulse_Width,msec)]
    Ventricle_Sensing1 -> Ventricle_Sensed2 [order 3] : [PB==1]
    DDDR_PaceA -> Ventricle_Sensing1 : [after(Pulse_Width,msec)]
    Ventricle_Sensing1 -> Ventricle_Sensed2 [order 2] : [VENT_CMP_DETECT == 1]
    DDDR_PaceV -> DDDR_charge : [after(Pulse_Width,msec)]
    DDDR_PaceV1 -> DDDR_charge : [after(Pulse_Width,msec)]
    Ventricle_Sensing1 -> DDDR_PaceV [order 1] : [after(AV_Delay-Pulse_Width,msec)]
  IDLE_STATE -> AOO [order 1] : [Mode == 0]
  AOO -> IDLE_STATE : [Mode ~= 0]
  IDLE_STATE -> AOOR [order 5] : [Mode == 4]
  AOOR -> IDLE_STATE : [Mode ~= 4]
  IDLE_STATE -> VVIR [order 8] : [Mode == 7]
  VVIR -> IDLE_STATE : [Mode ~= 7]
  (default) -> IDLE_STATE
  IDLE_STATE -> VVI [order 4] : [Mode == 3]
  IDLE_STATE -> AAI [order 3] : [Mode == 2]
  AAI -> IDLE_STATE : [Mode ~= 2]
  VVI -> IDLE_STATE : [Mode ~= 3]
  IDLE_STATE -> AAIR [order 7] : [Mode == 6]
  AAIR -> IDLE_STATE : [Mode ~= 6]
  IDLE_STATE -> VOOR [order 6] : [Mode == 5]
  VOOR -> IDLE_STATE : [Mode ~= 5]
  IDLE_STATE -> VOO [order 2] : [Mode == 1]
  VOO -> IDLE_STATE : [Mode ~= 1]
  IDLE_STATE -> DDDR [order 9] : [Mode == 8]
  DDDR -> IDLE_STATE : [Mode ~= 8]
  data: AMP input uint16; ATR_GND_CTRL output; ATR_PACE_CTRL output; PACE_CHARGE_CTRL output; PACE_GND_CTRL output; PACING_REF_PWM output; VENT_GND_CTRL output; VENT_PACE_CTRL output; Z_ATR_CTRL output; Z_VENT_CTRL output; LRL input; Pulse_Width input single; Mode input uint16; FRONTEND_CTRL output; VENT_CMP_DETECT input; ATR_CMP_DETECT input; SENSE_THRES input uint16; VENT_CMP_REF_PWM output; ATR_CMP_REF_PWM output; BLUE_LED output; RED_LED output; ARP input single; VRP input single; URL input uint16; Adapted_rate input; AV_Delay input; PB input
